simulink model "Fre_Synchron"  (Simulink 6.0)
settings: Solver=VariableStepDiscrete  StartTime=0.0  StopTime=.075  RelTol=1e-3
undefined symbols (not defined in the file or in its folder): Fre_offset_CDMA, Fre_Syn_CDMA
libraries: commchan2 x2, commdigbbndpm2 x2, dspsrcs4 x2, commseqgen2 x2, simulink x1, dspstat3 x1
settings Model: Creator=Administrator  LastModifiedBy=Hexingjian
settings OptimizationCC: InlineInvariantSignals=off  ExpressionDepthLimit=2147483647
settings DebuggingCC: SignalResolutionControl=UseLocalSettings  FcnCallInpInsideContextMsg=Use local settings  StateNameClashWarn=warning  StrictBusMsg=Warning
settings CodeAppCC: CustomSymbolStrType=$N$R$M

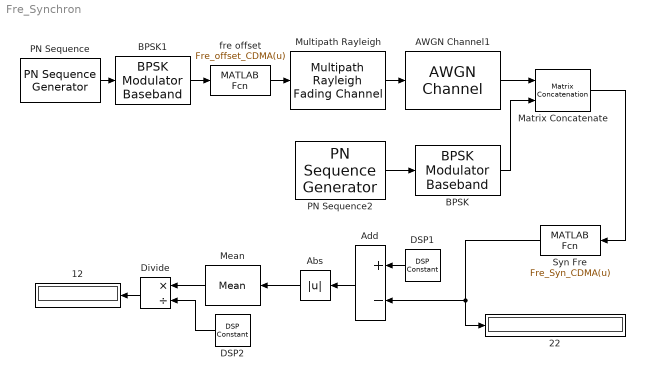
== system Fre_Synchron ==
  12 : Display
  22 : Display
  AWGN Channel1 : commchan2/AWGN Channel  SystemSampleTime=-1  seed=6724  noiseMode="Signal to noise ratio  (SNR)"  EbNodB=5  EsNodB=10  SNRdB=10  bitsPerSym=1  Ps=.5  Tsym=1e-6  variance=1
  Abs : Abs  Orientation=left
  Add : Sum  Orientation=left  Inputs=+-  OutScaling=2^-10
  BPSK : commdigbbndpm2/BPSK Modulator Baseband  SystemSampleTime=-1  Ph=0
  BPSK1 : commdigbbndpm2/BPSK Modulator Baseband  SystemSampleTime=-1  Ph=0
  DSP1 : dspsrcs4/DSP Constant  Orientation=left  SystemSampleTime=-1  Value=0.25  SampleMode=Discrete  discreteOutput=Sample-based  continuousOutput=Sample-based  sampTime=63e-6  framePeriod=256  dataType=Inherit from 'Constant value'  isSigned=on  wordLen=16  udDataType=sfix(16)  fracBitsMode=Best precision  numFracBits=15  InterpretAs1D=-inf  Ts=-inf  FramebasedOutput=-inf
  DSP2 : dspsrcs4/DSP Constant  Orientation=left  SystemSampleTime=-1  Value=0.25  SampleMode=Discrete  discreteOutput=Sample-based  continuousOutput=Sample-based  sampTime=63e-6  framePeriod=256  dataType=Inherit from 'Constant value'  isSigned=on  wordLen=16  udDataType=sfix(16)  fracBitsMode=Best precision  numFracBits=15  InterpretAs1D=-inf  Ts=-inf  FramebasedOutput=-inf
  Divide : Product  Orientation=left  Inputs=*/  OutScaling=2^-10
  Matrix Concatenate : simulink/Math Operations/Matrix Concatenation  numInports=2  catMethod=Vertical
  Mean : dspstat3/Mean  Orientation=left  DialogController=dspDDGCreate  DialogControllerArgs=DataTag0  run=on  reset_popup=None  roundingMode=Floor  overflowMode=off
  Multipath Rayleigh : commchan2/Multipath Rayleigh Fading Channel  SystemSampleTime=-1  seed=73
  PN Sequence : commseqgen2/PN Sequence Generator  poly=[6 5 0]  ini_sta=[0 0 0 0 0 1]  shift=0  Ts=1e-6  frameBased=on  sampPerFrame=63  reset=off
  PN Sequence2 : commseqgen2/PN Sequence Generator  poly=[6 5 0]  ini_sta=[0 0 0 0 0 1]  shift=0  Ts=1e-6  frameBased=on  sampPerFrame=63  reset=off
  Syn Fre : MATLABFcn  Orientation=left  MATLABFcn=Fre_Syn_CDMA(u)  Output1D=off
  fre offset : MATLABFcn  MATLABFcn=Fre_offset_CDMA(u)  Output1D=off
  wires:
  Multipath Rayleigh/1 -> AWGN Channel1/1
  AWGN Channel1/1 -> Matrix Concatenate/1
  PN Sequence/1 -> BPSK1/1
  BPSK1/1 -> fre offset/1
  BPSK/1 -> Matrix Concatenate/2
  PN Sequence2/1 -> BPSK/1
  fre offset/1 -> Multipath Rayleigh/1
  Matrix Concatenate/1 -> Syn Fre/1
  Add/1 -> Abs/1
  Abs/1 -> Mean/1
  Mean/1 -> Divide/1
  Divide/1 -> 12/1
  DSP1/1 -> Add/1
  DSP2/1 -> Divide/2
  Syn Fre/1 -> Add/2, 22/1
